simulink library "BeamStressLib"  (R2020a)
settings: Solver=VariableStepAuto  StartTime=0.0  StopTime=10.0  RelTol=1e-3
undefined symbols (not defined in the file): X, Y, Z
libraries: nesl_utility x16, sm_lib x9, sharedtransform x3
(part 2 of 2)

== matlab function BeamStressLib/Beam/MATLAB Function - Stress analysis ==
  data: F_A input; F_B input; stress_portA output; b input; h input; stress_portB output
function [stress_portA, stress_portB] = fcn(F_A, F_B, b, h)
%%%%%%%%%%%%%%%%%%%%%%%%%%%%%%%%%%%%%%%%%%%%%%%%%%%%%%%%%%%%%%%%%%%%%%%%%%%
% INPUTS:
%               F_A  = Forces and moments that act on the port A of the beam
%
%               F_A  = Forces and moments that act on the port A of the beam
%
%                 b  = Width of the beam (in x direction!).
%                      This is NOT strictly smaller than h.
%
%                 h  = Heigth of the beam (in y direction!).
%                      This is NOT strictly bigger than b.
%
%%%%%%%%%%%%%%%%%%%%%%%%%%%%%%%%%%%%%%%%%%%%%%%%%%%%%%%%%%%%%%%%%%%%%%%%%%%
% OUTPUTS:
%       stress_portA = Von Mises stress in the port A of the beam (vector with 9 elements).
%                      In particular
%                      - the 1st element (named A) is point with coordinate [+b/2 +h/2]
%                      - the 2nd element (named B) is point with coordinate [-b/2 +h/2]
%                      - the 3rd element (named C) is point with coordinate [-b/2 -h/2]
%                      - the 4th element (named D) is point with coordinate [+b/2 -h/2]
%                      - the 5th element (named E) is point with coordinate [  0  +h/2]
%                      - the 6th element (named F) is point with coordinate [-b/2   0 ]
%                      - the 7th element (named G) is point with coordinate [  0  -h/2]
%                      - the 8th element (named H) is point with coordinate [+b/2   0 ]
%                      - the 9th element (named I) is point with coordinate [  0    0 ]
%
%
%       stress_portB = Von Mises stress in the port A of the beam (vector with 9 elements).
%                      In particular
%                      - the 1st element (named A) is point with coordinate [+b/2 +h/2]
%                      - the 2nd element (named B) is point with coordinate [-b/2 +h/2]
%                      - the 3rd element (named C) is point with coordinate [-b/2 -h/2]
%                      - the 4th element (named D) is point with coordinate [+b/2 -h/2]
%                      - the 5th element (named E) is point with coordinate [  0  +h/2]
%                      - the 6th element (named F) is point with coordinate [-b/2   0 ]
%                      - the 7th element (named G) is point with coordinate [  0  -h/2]
%                      - the 8th element (named H) is point with coordinate [+b/2   0 ]
%                      - the 9th element (named I) is point with coordinate [  0    0 ]
%
%
% Cross section view of the beam.
%                                   ↑ y
%                                   |
%                                   |
%                  B               E|                A
%                   *---------------*---------------*            ----
%                   |               |               |               ↑
%                   |               |               |               |
%                   |               |               |               |
%                   |               |               |        x      |
%                 F *               *---------------* H ----→      h
%                   |              I                |               |
%                   |                               |               |
%                   |                               |               |
%                   |                               |               ↓
%                   *---------------*---------------*            ----
%                  C               G                 D
%
%                   |                               |
%                   |                               |
%                   ⇤--------------b---------------⇥
%
%
%
%%%%%%%%%%%%%%%%%%%%%%%%%%%%%%%%%%%%%%%%%%%%%%%%%%%%%%%%%%%%%%%%%%%%%%%%%%%
% HYPOTESIS and NOTES:
%
%  0) We compute stresses only for generic beams with rectangular (or squared)
%     cross section.
%  1) The stress of this routine are check with NX Nastran FEM software by
%     the author using a 1D beam model with generic loading (lumped force
%     and moments, in ordet to validate the goodness of the results.
%     The present routine give results in good agreement with sthe FEM model.
%  
%%%%%%%%%%%%%%%%%%%%%%%%%%%%%%%%%%%%%%%%%%%%%%%%%%%%%%%%%%%%%%%%%%%%%%%%%%%
% Author: Alberto Mora, (STIIMA - CNR)   http://www.stiima.cnr.it/en/
% Date:   26/05/2020
%%%%%%%%%%%%%%%%%%%%%%%%%%%%%%%%%%%%%%%%%%%%%%%%%%%%%%%%%%%%%%%%%%%%%%%%%%%
% REVISION:
%       v0.0 First release
%%%%%%%%%%%%%%%%%%%%%%%%%%%%%%%%%%%%%%%%%%%%%%%%%%%%%%%%%%%%%%%%%%%%%%%%%%% 
%% FIRST CALCULATIONS
                                                                            
% Let compute info about the beam cross section
Ix = b*h^3/12;                                                              % Inertia along X axis of the cross section [e.g. m^4]
Iy = b^3*h/12;                                                              % Inertia along Y axis of the cross section [e.g. m^4]
A = b*h;                                                                    % Cross section [e.g. m^2]

% For shear stress in non-circular (rectangular) beams we have to find the
% smaller and bigger edge of the cross section. Then we have to check if
% the longer edge (aa) is along x axis (so equal to b) or along y axis (so
% equal to h).
aa=max([b h]);
bb=min([b h]);
aa_is_along_x_axis = aa==b;

Pa_to_MPa = 10^-6;                                                          % Convert Pa to MPa (always used in mechanical engineering)

%% STRESS PORT A (lower, the one attacched at the origin)

% PORT A. Since we are considering force applied to the port A, looking to the left-end
% of the beam we have to change the sign. Divide the loads vector into force and
% moment vector.
F=-F_A(1:3);
M=-F_A(4:6);



% Point A    [+b/2 +h/2]
sigma_A_Mx = M(1)*( h/2)/Ix;
sigma_A_My = M(2)*(-b/2)/Iy;
sigma_A_z = F(3)/A;
sigma_A_von_mises = abs(sigma_A_Mx + sigma_A_My + sigma_A_z);               % Since on A, B, C, D point we don't have shear stress,
                                                                            % this value is already the von-mises (simple a combination
                                                                            % of normal stresses)

% Point B    [-b/2 +h/2]
sigma_B_Mx = M(1)*( h/2)/Ix;
sigma_B_My = M(2)*( b/2)/Iy;
sigma_B_z = F(3)/A;
sigma_B_von_mises = abs(sigma_B_Mx + sigma_B_My + sigma_B_z);

% Point C    [-b/2 -h/2]
sigma_C_Mx = M(1)*(-h/2)/Ix;
sigma_C_My = M(2)*( b/2)/Iy;
sigma_C_z = F(3)/A;
sigma_C_von_mises = abs(sigma_C_Mx + sigma_C_My + sigma_C_z);

% Point D    [+b/2 -h/2]
sigma_D_Mx = M(1)*(-h/2)/Ix;
sigma_D_My = M(2)*(-b/2)/Iy;
sigma_D_z = F(3)/A;
sigma_D_von_mises = abs(sigma_D_Mx + sigma_D_My + sigma_D_z);

% Point E    [ 0 +h/2 ]
if aa_is_along_x_axis==true
    % Long edge along X -> on E and G we have higher stresses (while on F and H we have lower stresses)
    coeff_alpha =  2.94+2.744/(aa/bb+0.482);                                % Better approximation than the traditional   (3.0+1.8*bb/aa)    of the Manuale di meccanica. Found numerically by creating a new fitting function.
    tau_E_Mz = coeff_alpha * (- M(3)/(aa*bb^2));                            % Torque stress, see Manuale di meccanica Hoepli, page 981 H-100
else
    % Long edge along Y -> on E we have lower stresses
    tau_E_Mz = (2.2+2.6*bb/aa) * (- M(3)/(aa*bb^2));                        % Torque stress, see Manuale di meccanica Hoepli, page 981 H-100
end
tau_E_Fx = 1.5 * F(1)/A;                                                    % Shear stress on X, see Manuale di meccanica Hoepli, page 974 H-93 H-100
tau_E_Fy = 0;                                                               % Shear stress on Y 
sigma_E_Mx = M(1)*( h/2)/Ix;
sigma_E_My = 0;
sigma_E_z = F(3)/A;
sigma_E_von_mises = (  (sigma_E_Mx+sigma_E_My+sigma_E_z)^2 + 3*(tau_E_Fx+tau_E_Fy+tau_E_Mz)^2  )^0.5;


% Point F    [ -b/2   0 ]
if aa_is_along_x_axis==true
    % Long edge along X -> on F we have lower stresses
    tau_F_Mz = (2.2+2.6*bb/aa) * (- M(3)/(aa*bb^2));
else
    % Long edge along Y -> on F we have higher stresses
    coeff_alpha =  2.94+2.744/(aa/bb+0.482);
    tau_F_Mz = coeff_alpha * (- M(3)/(aa*bb^2));
end
tau_F_Fx = 0;
tau_F_Fy = 1.5 * F(2)/A;
sigma_F_Mx = 0;
sigma_F_My = M(2)*( b/2)/Iy;
sigma_F_z = F(3)/A;
sigma_F_von_mises = (  (sigma_F_Mx+sigma_F_My+sigma_F_z)^2 + 3*(tau_F_Fx+tau_F_Fy+tau_F_Mz)^2  )^0.5;



% Point G    [ 0 -h/2 ]
if aa_is_along_x_axis==true
    % Long edge along X -> on G we have higher stresses
    coeff_alpha =  2.94+2.744/(aa/bb+0.482);
    tau_G_Mz = coeff_alpha * (  M(3)/(aa*bb^2));
else
    % Long edge along Y -> on G we have lower stresses
    tau_G_Mz = (2.2+2.6*bb/aa) * (  M(3)/(aa*bb^2));
end
tau_G_Fx = 1.5 * F(1)/A;
tau_G_Fy = 0;
sigma_G_Mx = M(1)*(-h/2)/Ix;
sigma_G_My = 0;
sigma_G_z = F(3)/A;
sigma_G_von_mises = (  (sigma_G_Mx+sigma_G_My+sigma_G_z)^2 + 3*(tau_G_Fx+tau_G_Fy+tau_G_Mz)^2  )^0.5;


% Point H    [ +b/2   0 ]
if aa_is_along_x_axis==true
    % Long edge along X -> on H we have lower stresses
    tau_H_Mz = (2.2+2.6*bb/aa) * (  M(3)/(aa*bb^2));
else
    % Long edge along Y -> on H we have higher stresses
    coeff_alpha =  2.94+2.744/(aa/bb+0.482);
    tau_H_Mz = coeff_alpha * (  M(3)/(aa*bb^2));
end
tau_H_Fx = 0;
tau_H_Fy = 1.5 * F(2)/A;
sigma_H_Mx = 0;
sigma_H_My = M(2)*(-b/2)/Iy;
sigma_H_z = F(3)/A;
sigma_H_von_mises = (  (sigma_H_Mx+sigma_H_My+sigma_H_z)^2 + 3*(tau_H_Fx+tau_H_Fy+tau_H_Mz)^2  )^0.5;


% Point I    [ 0   0 ]
% This is the hardest point. We cannot use simple von-mises formula for monoaxial stress and shear in 1 direction as done in the previous points.
% We have to compute the stress tensor, then extract the principal stresses (roots of the Mohr's circle), and then use the generalized
% formula of Von-Mises for a generic triaxial stress state.
tau_I_Mz = 0;                                                               % Torsion is null at the center of the beam, there is only shear on both directions x and y and there is also compression
tau_I_Fx = 1.5 * F(1)/A;
tau_I_Fy = 1.5 * F(2)/A;
sigma_I_Mx = 0;
sigma_I_My = 0;
sigma_I_z = F(3)/A;
tensor_stress_I = [   0          0      tau_I_Fx;                           % Let compute the stress tensor
                      0          0      tau_I_Fy;
                 tau_I_Fx   tau_I_Fy  sigma_I_z ];
principal_stress = eig(tensor_stress_I);                                    % Principal stress (zero of the Mohr circle)
sigma_I_von_mises = real(  sqrt( ((principal_stress(1)-principal_stress(2))^2  +...
                                  (principal_stress(2)-principal_stress(3))^2  +...
                                  (principal_stress(1)-principal_stress(3))^2 )/2   ) ) ;% Von mises equivalent stress (for triaxial loading).
                                                                            % Keep only real part (small problems of numerical computations that leads to a very small imaginary component)


stress_portA = [sigma_A_von_mises
                sigma_B_von_mises
                sigma_C_von_mises
                sigma_D_von_mises
                sigma_E_von_mises
                sigma_F_von_mises
                sigma_G_von_mises
                sigma_H_von_mises
                sigma_I_von_mises]*Pa_to_MPa;


%% STRESS PORT B (upper one, the one with offset dz=+length)

% PORT B. Since we are considering force applied to the port B, looking to the right-end
% of the beam we keep sign as default. Divide the loads vector into force and
% moment vector.
F=F_B(1:3);
M=F_B(4:6);


% Point A    [+b/2 +h/2]
sigma_A_Mx = M(1)*( h/2)/Ix;
sigma_A_My = M(2)*(-b/2)/Iy;
sigma_A_z = F(3)/A;
sigma_A_von_mises = abs(sigma_A_Mx + sigma_A_My + sigma_A_z);               % Since on A, B, C, D point we don't have shear stress,
                                                                            % this value is already the von-mises (simple a combination
                                                                            % of normal stresses)

% Point B    [-b/2 +h/2]
sigma_B_Mx = M(1)*( h/2)/Ix;
sigma_B_My = M(2)*( b/2)/Iy;
sigma_B_z = F(3)/A;
sigma_B_von_mises = abs(sigma_B_Mx + sigma_B_My + sigma_B_z);

% Point C    [-b/2 -h/2]
sigma_C_Mx = M(1)*(-h/2)/Ix;
sigma_C_My = M(2)*( b/2)/Iy;
sigma_C_z = F(3)/A;
sigma_C_von_mises = abs(sigma_C_Mx + sigma_C_My + sigma_C_z);

% Point D    [+b/2 -h/2]
sigma_D_Mx = M(1)*(-h/2)/Ix;
sigma_D_My = M(2)*(-b/2)/Iy;
sigma_D_z = F(3)/A;
sigma_D_von_mises = abs(sigma_D_Mx + sigma_D_My + sigma_D_z);

% Point E    [ 0 +h/2 ]
if aa_is_along_x_axis==true
    % Long edge along X -> on E and G we have higher stresses (while on F and H we have lower stresses)
    coeff_alpha =  2.94+2.744/(aa/bb+0.482);                                % Better approximation than the traditional   (3.0+1.8*bb/aa)    of the Manuale di meccanica. Found numerically by creating a new fitting function.
    tau_E_Mz = coeff_alpha * (- M(3)/(aa*bb^2));                            % Torque stress, see Manuale di meccanica Hoepli, page 981 H-100
else
    % Long edge along Y -> on E we have lower stresses
    tau_E_Mz = (2.2+2.6*bb/aa) * (- M(3)/(aa*bb^2));                        % Torque stress, see Manuale di meccanica Hoepli, page 981 H-100
end
tau_E_Fx = 1.5 * F(1)/A;                                                    % Shear stress on X, see Manuale di meccanica Hoepli, page 974 H-93 H-100
tau_E_Fy = 0;                                                               % Shear stress on Y 
sigma_E_Mx = M(1)*( h/2)/Ix;
sigma_E_My = 0;
sigma_E_z = F(3)/A;
sigma_E_von_mises = (  (sigma_E_Mx+sigma_E_My+sigma_E_z)^2 + 3*(tau_E_Fx+tau_E_Fy+tau_E_Mz)^2  )^0.5;


% Point F    [ -b/2   0 ]
if aa_is_along_x_axis==true
    % Long edge along X -> on F we have lower stresses
    tau_F_Mz = (2.2+2.6*bb/aa) * (- M(3)/(aa*bb^2));
else
    % Long edge along Y -> on F we have higher stresses
    coeff_alpha =  2.94+2.744/(aa/bb+0.482);
    tau_F_Mz = coeff_alpha * (- M(3)/(aa*bb^2));
end
tau_F_Fx = 0;
tau_F_Fy = 1.5 * F(2)/A;
sigma_F_Mx = 0;
sigma_F_My = M(2)*( b/2)/Iy;
sigma_F_z = F(3)/A;
sigma_F_von_mises = (  (sigma_F_Mx+sigma_F_My+sigma_F_z)^2 + 3*(tau_F_Fx+tau_F_Fy+tau_F_Mz)^2  )^0.5;



% Point G    [ 0 -h/2 ]
if aa_is_along_x_axis==true
    % Long edge along X -> on G we have higher stresses
    coeff_alpha =  2.94+2.744/(aa/bb+0.482);
    tau_G_Mz = coeff_alpha * (  M(3)/(aa*bb^2));
else
    % Long edge along Y -> on G we have lower stresses
    tau_G_Mz = (2.2+2.6*bb/aa) * (  M(3)/(aa*bb^2));
end
tau_G_Fx = 1.5 * F(1)/A;
tau_G_Fy = 0;
sigma_G_Mx = M(1)*(-h/2)/Ix;
sigma_G_My = 0;
sigma_G_z = F(3)/A;
sigma_G_von_mises = (  (sigma_G_Mx+sigma_G_My+sigma_G_z)^2 + 3*(tau_G_Fx+tau_G_Fy+tau_G_Mz)^2  )^0.5;


% Point H    [ +b/2   0 ]
if aa_is_along_x_axis==true
    % Long edge along X -> on H we have lower stresses
    tau_H_Mz = (2.2+2.6*bb/aa) * (  M(3)/(aa*bb^2));
else
    % Long edge along Y -> on H we have higher stresses
    coeff_alpha =  2.94+2.744/(aa/bb+0.482);
    tau_H_Mz = coeff_alpha * (  M(3)/(aa*bb^2));
end
tau_H_Fx = 0;
tau_H_Fy = 1.5 * F(2)/A;
sigma_H_Mx = 0;
sigma_H_My = M(2)*(-b/2)/Iy;
sigma_H_z = F(3)/A;
sigma_H_von_mises = (  (sigma_H_Mx+sigma_H_My+sigma_H_z)^2 + 3*(tau_H_Fx+tau_H_Fy+tau_H_Mz)^2  )^0.5;


% Point I    [ 0   0 ]
% This is the hardest point. We cannot use simple von-mises formula for monoaxial stress and shear in 1 direction as done in the previous points.
% We have to compute the stress tensor, then extract the principal stresses (roots of the Mohr's circle), and then use the generalized
% formula of Von-Mises for a generic triaxial stress state.
tau_I_Mz = 0;                                                               % Torsion is null at the center of the beam, there is only shear on both directions x and y and there is also compression
tau_I_Fx = 1.5 * F(1)/A;
tau_I_Fy = 1.5 * F(2)/A;
sigma_I_Mx = 0;
sigma_I_My = 0;
sigma_I_z = F(3)/A;
tensor_stress_I = [   0          0      tau_I_Fx;                           % Let compute the stress tensor
                      0          0      tau_I_Fy;
                 tau_I_Fx   tau_I_Fy  sigma_I_z ];
principal_stress = eig(tensor_stress_I);                                    % Principal stress (zero of the Mohr circle)
sigma_I_von_mises = real(  sqrt( ((principal_stress(1)-principal_stress(2))^2  +...
                                  (principal_stress(2)-principal_stress(3))^2  +...
                                  (principal_stress(1)-principal_stress(3))^2 )/2   ) ) ;% Von mises equivalent stress (for triaxial loading).
                                                                            % Keep only real part (small problems of numerical computations that leads to a very small imaginary component)


stress_portB = [sigma_A_von_mises
                sigma_B_von_mises
                sigma_C_von_mises
                sigma_D_von_mises
                sigma_E_von_mises
                sigma_F_von_mises
                sigma_G_von_mises
                sigma_H_von_mises
                sigma_I_von_mises]*Pa_to_MPa;
